simulink model "yaw_test"  (R2017b)
settings: Solver=VariableStepAuto  StartTime=0.0  StopTime=5  RelTol=1e-3
libraries: NLGCToolbox x2
settings Model: Creator=hoang  LastModifiedBy=hoang

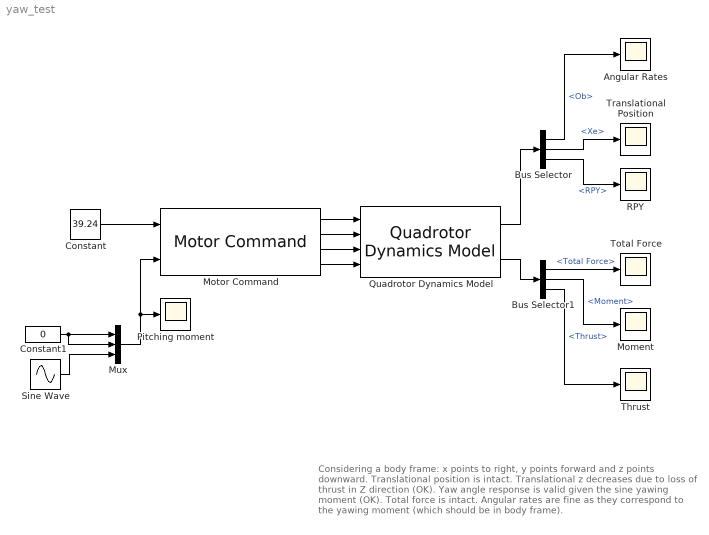
== system yaw_test ==
  note: Considering a body frame: x points to right, y points forward and z points downward.
      | Translational position is intact.
      | Translational z decreases due to loss of thrust in Z direction (OK).
      | Yaw angle response is valid given the sine yawing moment (OK).
      | Total force is intact.
      | Angular rates are fine as they correspond to the yawing moment (which should be in body frame).
  Angular Rates : Scope
  Bus Selector : BusSelector  OutputSignals=Ob,Xe,RPY
  Bus Selector1 : BusSelector  OutputSignals=Total Force,Moment,Thrust
  Constant : Constant  Value=39.24
  Constant1 : Constant  Value=0
  Moment : Scope
  Motor Command : NLGCToolbox/Motor Command  quadrotor=quad
      settings: SourceProductName=Thinh - NLGC for Quadrotor
  Mux : Mux  Inputs=3
  Pitching moment : Scope
  Quadrotor Dynamics Model : NLGCToolbox/Quadrotor Dynamics Model  xinit=[0 0 -4]  quadrotor=quad
      settings: SourceProductName=Thinh - NLGC for Quadrotor
  RPY : Scope
  Sine Wave : Sin  Amplitude=0.005  Frequency=2*pi/5  SampleTime=0
  Thrust : Scope
  Total Force : Scope
  Translational Position : Scope
  wires:
  Motor Command/1 -> Quadrotor Dynamics Model/1
  Motor Command/2 -> Quadrotor Dynamics Model/2
  Motor Command/3 -> Quadrotor Dynamics Model/3
  Motor Command/4 -> Quadrotor Dynamics Model/4
  Constant/1 -> Motor Command/1
  Quadrotor Dynamics Model/1 -> Bus Selector/1
  Bus Selector/2 -> Translational Position/1  "<Xe>"
  Bus Selector/3 -> RPY/1  "<RPY>"
  Quadrotor Dynamics Model/2 -> Bus Selector1/1
  Bus Selector1/1 -> Total Force/1  "<Total Force>"
  Bus Selector1/2 -> Moment/1  "<Moment>"
  Mux/1 -> Pitching moment/1, Motor Command/2
  Bus Selector1/3 -> Thrust/1  "<Thrust>"
  Constant1/1 -> Mux/2, Mux/1
  Bus Selector/1 -> Angular Rates/1  "<Ob>"
  Sine Wave/1 -> Mux/3
